simulink model "WindPrototipeN"  (R2019b)
settings: Solver=ode23s  StartTime=0.0  StopTime=Ts  FixedStep=2  RelTol=5
values from neighbouring files (symbols this model uses):
  c1 = 0.51763    [matlab.mat]
  c2 = 116    [matlab.mat]
  c3 = 0.4    [matlab.mat]
  c4 = 5    [matlab.mat]
  c5 = 21    [matlab.mat]
  c6 = 0.006795    [matlab.mat]
  Tp = 2e-05    [matlab.mat]
undefined symbols (not defined in the file or in its folder): Cogent, DiscIntNeverNeededParam, Ion, Kepware, Lithium, localhost, sigbuilder_block
libraries: powerlib x266, powerlib_extras x83, simulink x30, powerlib_meascontrol x13, opclib x11, sldrtlib x8, electricdrivelib x3
(part 4 of 9)

== system WindPrototipeN/Дом 2/ПОТРЕБИТЕЛЬ1 ==
  1000 Вт1 : powerlib/Elements/Three-Phase Parallel RLC Load  LConnTagsString=A|B|C  Configuration=Y (grounded)  NominalVoltage=385  Vabc=[1e3 1e3 1e3]  Vabcp=[1e3 1e3 1e3]  NominalFrequency=50  UnbalancedPower=off  ActivePower=1000  InductivePower=0  CapacitivePower=0  Pabc=[10e3 9e3 11e3]  QLabc=[100 90 110]  QCabc=[100 90 110]  Pabcp=[10e3 9e3 11e3]  QLabcp=[100 90 110]  QCabcp=[100 90 110]  Measurements=None  LoadType=constant Z
      settings: SourceProductName=Simscape Electrical
  1500 Вт1 : powerlib/Elements/Three-Phase Parallel RLC Load  LConnTagsString=A|B|C  Configuration=Y (grounded)  NominalVoltage=385  Vabc=[1e3 1e3 1e3]  Vabcp=[1e3 1e3 1e3]  NominalFrequency=50  UnbalancedPower=off  ActivePower=1000  InductivePower=0  CapacitivePower=0  Pabc=[10e3 9e3 11e3]  QLabc=[100 90 110]  QCabc=[100 90 110]  Pabcp=[10e3 9e3 11e3]  QLabcp=[100 90 110]  QCabcp=[100 90 110]  Measurements=None  LoadType=constant Z
      settings: SourceProductName=Simscape Electrical
  500 Вт (1)1 : powerlib/Elements/Three-Phase Parallel RLC Load  LConnTagsString=A|B|C  Configuration=Y (grounded)  NominalVoltage=385  Vabc=[1e3 1e3 1e3]  Vabcp=[1e3 1e3 1e3]  NominalFrequency=50  UnbalancedPower=off  ActivePower=500  InductivePower=0  CapacitivePower=0  Pabc=[10e3 9e3 11e3]  QLabc=[100 90 110]  QCabc=[100 90 110]  Pabcp=[10e3 9e3 11e3]  QLabcp=[100 90 110]  QCabcp=[100 90 110]  Measurements=None  LoadType=constant Z
      settings: SourceProductName=Simscape Electrical
  500 Вт (2)1 : powerlib/Elements/Three-Phase Parallel RLC Load  LConnTagsString=A|B|C  Configuration=Y (grounded)  NominalVoltage=385  Vabc=[1e3 1e3 1e3]  Vabcp=[1e3 1e3 1e3]  NominalFrequency=50  UnbalancedPower=off  ActivePower=500  InductivePower=0  CapacitivePower=0  Pabc=[10e3 9e3 11e3]  QLabc=[100 90 110]  QCabc=[100 90 110]  Pabcp=[10e3 9e3 11e3]  QLabcp=[100 90 110]  QCabcp=[100 90 110]  Measurements=None  LoadType=constant Z
      settings: SourceProductName=Simscape Electrical
  BL : powerlib/Measurements/Three-Phase V-I Measurement  VoltageMeasurement=phase-to-ground  SetLabelV=on  LabelV=Vabc_BL_ex  Vpu=off  VpuLL=off  CurrentMeasurement=yes  SetLabelI=on  LabelI=Iabc_BL_ex  Ipu=off  Pbase=100e6  Vbase=500e3  OutputType=Magnitude  PhasorSimulation=off  PSBequivalent=0
      settings: SourceProductName=Simscape Electrical
  Subsystem1 : Subsystem
  Three-Phase Breaker10 : powerlib/Elements/Three-Phase Breaker  InitialState=open  SwitchA=on  SwitchB=on  SwitchC=on  SwitchTimes=[6 7]  External=on  BreakerResistance=0.001  SnubberResistance=1e6  SnubberCapacitance=inf  Measurements=None
      settings: SourceProductName=Simscape Electrical
  Three-Phase Breaker11 : powerlib/Elements/Three-Phase Breaker  InitialState=open  SwitchA=on  SwitchB=on  SwitchC=on  SwitchTimes=[7 10]  External=on  BreakerResistance=0.001  SnubberResistance=1e6  SnubberCapacitance=inf  Measurements=None
      settings: SourceProductName=Simscape Electrical
  Three-Phase Breaker8 : powerlib/Elements/Three-Phase Breaker  InitialState=open  SwitchA=on  SwitchB=on  SwitchC=on  SwitchTimes=[0 5]  External=on  BreakerResistance=0.001  SnubberResistance=1e6  SnubberCapacitance=inf  Measurements=None
      settings: SourceProductName=Simscape Electrical
  Three-Phase Breaker9 : powerlib/Elements/Three-Phase Breaker  InitialState=open  SwitchA=on  SwitchB=on  SwitchC=on  SwitchTimes=[2 5]  External=on  BreakerResistance=0.001  SnubberResistance=1e6  SnubberCapacitance=inf  Measurements=None
      settings: SourceProductName=Simscape Electrical
  Блок измерений : powerlib/Measurements/Three-Phase V-I Measurement  VoltageMeasurement=phase-to-ground  SetLabelV=off  LabelV=V1  Vpu=off  VpuLL=off  CurrentMeasurement=yes  SetLabelI=off  LabelI=I1  Ipu=off  Pbase=5.5e3  Vbase=385  OutputType=Magnitude  PhasorSimulation=off  PSBequivalent=0
      settings: SourceProductName=Simscape Electrical
  Терминал нагрузки : Scope  NumInputPorts=2
  A : PMIOPort  Side=Left
  B : PMIOPort  Port=2  Side=Left
  C : PMIOPort  Port=3  Side=Left
  tag scope: Iload_ex=global, Load2Home1=global, Load2Home2=global, Load2Home3=global, Load2Home4=global, Vload_ex=global
  wires:
  Блок измерений/1 -> [Vload_ex], Терминал нагрузки/1  "Напряжение, В"
  Блок измерений/2 -> [Iload_ex], Терминал нагрузки/2  "Сила тока, А"
  Subsystem1/3(Out3) -> [Load2Home3], Three-Phase Breaker10/1
  Subsystem1/1(Out1) -> [Load2Home1], Three-Phase Breaker8/1
  Subsystem1/4(Out4) -> [Load2Home4], Three-Phase Breaker11/1
  Subsystem1/2(Out2) -> [Load2Home2], Three-Phase Breaker9/1
  connections:
  BL/RConn1 -- Блок измерений/LConn1
  BL/RConn2 -- Блок измерений/LConn2
  BL/RConn3 -- Блок измерений/LConn3
  BL/LConn1 -- A/RConn1
  BL/LConn2 -- B/RConn1
  C/RConn1 -- BL/LConn3
  Three-Phase Breaker10/RConn1 -- Three-Phase Breaker9/RConn1 -- Блок измерений/RConn1 -- Three-Phase Breaker8/RConn1 -- Three-Phase Breaker11/RConn1
  Three-Phase Breaker10/RConn2 -- Three-Phase Breaker9/RConn2 -- Three-Phase Breaker8/RConn2 -- Блок измерений/RConn2 -- Three-Phase Breaker11/RConn2
  Three-Phase Breaker10/RConn3 -- Three-Phase Breaker9/RConn3 -- Three-Phase Breaker8/RConn3 -- Блок измерений/RConn3 -- Three-Phase Breaker11/RConn3
  500 Вт (1)1/LConn3 -- Three-Phase Breaker8/LConn3
  500 Вт (2)1/LConn2 -- Three-Phase Breaker9/LConn2
  1000 Вт1/LConn2 -- Three-Phase Breaker10/LConn2
  1500 Вт1/LConn3 -- Three-Phase Breaker11/LConn3
  1500 Вт1/LConn2 -- Three-Phase Breaker11/LConn2
  500 Вт (2)1/LConn1 -- Three-Phase Breaker9/LConn1
  1000 Вт1/LConn3 -- Three-Phase Breaker10/LConn3
  500 Вт (1)1/LConn2 -- Three-Phase Breaker8/LConn2
  1000 Вт1/LConn1 -- Three-Phase Breaker10/LConn1
  500 Вт (2)1/LConn3 -- Three-Phase Breaker9/LConn3
  1500 Вт1/LConn1 -- Three-Phase Breaker11/LConn1
  500 Вт (1)1/LConn1 -- Three-Phase Breaker8/LConn1

== system WindPrototipeN/Дом 2/СОЛНЕЧНЫЕ ПАНЕЛИ1 ==
  note: boost
  Солнечная радиация : Inport
  11*2=666 V : Subsystem
  FW Diode1 : powerlib/Power Electronics/Diode  Ron=0.01  Lon=0  Vf=0.8  IC=0  UseSnubber=off  Rs=100  Cs=0.1e-6  Measurements=off
      settings: SourceProductName=Simscape Electrical
  Gain : Gain  Gain=4732*2/1000
  IL1 : powerlib/Measurements/Current Measurement  PhasorSimulation=off  OutputType=Complex  PSBequivalent=0
      settings: SourceProductName=Simscape Electrical
  Mean Value1 : powerlib_extras/Measurements/Mean Value  Period=0.0045
      settings: SourceProductName=Simscape Electrical  SourceProductBaseCode=PS
  Mux : Mux  Inputs=2
  Product6 : Product  RndMeth=Zero
  Vdc2 : powerlib/Measurements/Voltage Measurement  Tag=PoWeRsYsTeMmEaSuReMeNt  PhasorSimulation=off  OutputType=Magnitude  PSBequivalent=0
      settings: SourceProductName=Simscape Electrical
  Мощность СП1 : Scope
  Мощность СП2 : Scope
  Мощность СП3_2 : Scope
  Мощность СП_2 : Scope
  Терминал данных параметров солнечной панели2 : Scope  NumInputPorts=4
  + : PMIOPort  Side=Right
  - : PMIOPort  Port=2  Side=Right
  Sp : Outport  VectorParamsAs1DForOutWhenUnconnected=off
  tag scope: Scur_ex=global, Sp_ex=global, Svol_ex=global
  wires:
  Vdc2/1 -> [Svol_ex], Мощность СП2/1, Терминал данных параметров солнечной панели2/4, Product6/1  "Напряжение, В"
  Product6/1 -> Mux/2, Sp/1, Терминал данных параметров солнечной панели2/2, [Sp_ex]  "Выходная мощность СЭУ, Вт"
  Gain/1 -> Mux/1, Терминал данных параметров солнечной панели2/1  "Интенсивность солнечной радиации, Вт/м2"
  Mux/1 -> Мощность СП_2/1
  Mean Value1/1 -> Product6/2
  IL1/1 -> Терминал данных параметров солнечной панели2/3, Mean Value1/1, [Scur_ex], Мощность СП1/1  "Сила тока, А"
  Солнечная радиация/1 -> Gain/1, Мощность СП3_2/1, 11*2=666 V/1(In1)
  connections:
  11*2=666 V/RConn2 -- Vdc2/LConn2 -- -/RConn1
  +/RConn1 -- IL1/RConn1
  11*2=666 V/RConn1 -- FW Diode1/LConn1 -- Vdc2/LConn1
  IL1/LConn1 -- FW Diode1/RConn1

== system WindPrototipeN/Дом 3/DC//AC 220В1 ==
  LC Фильтр : Subsystem
  PWM IGBT Inverter1 : powerlib/Power Electronics/Universal Bridge  Arms=3  SnubberResistance=5000  SnubberCapacitance=inf  Device=IGBT / Diodes  Ron=1e-3  Lon=0  ForwardVoltages="[  0.0  0.0  ]"  ForwardVoltage=.8  GTOparameters=[ 1e-6 ,1e-6 ]  IGBTparameters=[ 1e-6 , 2e-6 ]  Measurements=Device currents  Measurements_2=None  converterType=Rectifier
      settings: SourceProductName=Simscape Electrical
  Инвертор DC/AC : Subsystem
  Терминал инвертора : Scope  NumInputPorts=2
  A : PMIOPort  Side=Right
  B : PMIOPort  Port=2  Side=Right
  C : PMIOPort  Port=3  Side=Right
  + IGBT1 : PMIOPort  Port=4  Side=Left
  - IGBT1 : PMIOPort  Port=5  Side=Left
  wires:
  Инвертор DC/AC/3(Pulses) -> PWM IGBT Inverter1/1
  Инвертор DC/AC/1(VL) -> Терминал инвертора/1  "Напряжение на входе, В"
  Инвертор DC/AC/2(Vp) -> Терминал инвертора/2  "Напряжение от преобразователя, В"
  connections:
  LC Фильтр/LConn1 -- PWM IGBT Inverter1/LConn1
  LC Фильтр/RConn3 -- C/RConn1 -- Инвертор DC/AC/LConn1
  Инвертор DC/AC/LConn2 -- B/RConn1 -- LC Фильтр/RConn2
  LC Фильтр/RConn1 -- A/RConn1 -- Инвертор DC/AC/LConn3
  LC Фильтр/LConn3 -- PWM IGBT Inverter1/LConn3
  LC Фильтр/LConn2 -- PWM IGBT Inverter1/LConn2
  + IGBT1/RConn1 -- PWM IGBT Inverter1/RConn1
  - IGBT1/RConn1 -- PWM IGBT Inverter1/RConn2

== system WindPrototipeN/Дом 3/DC//DC ПРЕОБРАЗОВАТЕЛЬ ВЭУ1 ==
  Add : Sum
  CBus : powerlib/Elements/Series RLC Branch  LConnTagsString=__new0  RConnTagsString=__new0  BranchType=RC  Resistance=0.2  Inductance=1e-3  SetiL0=off  InitialCurrent=0  Capacitance=7500e-6  Setx0=on  InitialVoltage=100  Measurements=None
      settings: SourceProductName=Simscape Electrical
  Chopper : Subsystem  mask(SPSdrives Converter){SnubberResistance=10e3, SnubberCapacitance=inf, Ron=1e-3, ForwardVoltages=[1.3,1.3], IGBTParameters=[0,0], converterType=Inverter}
      mask prompts: SnubberResistance "Snubber resistance Rs (Ohms):"; SnubberCapacitance "Snubber capacitance Cs (F):"; Ron "Ron (Ohms):"; ForwardVoltages "Forward voltages [Device Vf(V), Diode Vd (V)]"; IGBTParameters "[Tf(s), Tt(s)]:"; converterType "Converter type:"
      mask help: This model implements an average-value buck converter."Duty Cycle" contains the duty cycle of the internal IGBT device.
      mask TypeOptions converterType: Rectifier | Inverter
      mask Display: plot(0,0,100,100,[39 39 23.8],[71 28 28],[44 56 49.6 56 52.8 56 61 61],[39.2 33.6 32.8 33.6 40.8 33.6 30 12.4],[44 44 44 61 61],[28 71 60 66.4 90],[75 67 83 75 67 83 75 75],[54 42 42 54 54 54 54 66],[61 75 75],[24 24 42],[75 75 61],[66,76,76])
  Constant : Constant  Value=100
  Current controller DISCRETE1 : Subsystem  mask(PI controller){Kp=0.0005, Ki=0.15, Ts=20e-6}
      mask prompts: Kp "Proportional gain (Kp)"; Ki "Integral gain (Ki)"; Ts "Sample time (s) :"
      mask help: Proportional-Integral Speed Controller
      mask Display: plot(0,0,100,100,[35,35,65],[70,30,30],[35,65],[45,60])
  Current controller DISCRETE2 : Subsystem  mask(PI controller){Kp=0.0005, Ki=0.15, Ts=20e-6}
      mask prompts: Kp "Proportional gain (Kp)"; Ki "Integral gain (Ki)"; Ts "Sample time (s) :"
      mask help: Proportional-Integral Speed Controller
      mask Display: plot(0,0,100,100,[35,35,65],[70,30,30],[35,65],[45,60])
  Duty Cycles : Subsystem
  IL2 : powerlib/Measurements/Current Measurement  PhasorSimulation=off  OutputType=Complex  PSBequivalent=0
      settings: SourceProductName=Simscape Electrical
  IL4 : powerlib/Measurements/Current Measurement  PhasorSimulation=off  OutputType=Complex  PSBequivalent=0
      settings: SourceProductName=Simscape Electrical
  L : powerlib/Elements/Series RLC Branch  LConnTagsString=__new0  RConnTagsString=__new0  BranchType=L  Resistance=0.3  Inductance=500e-6  SetiL0=off  InitialCurrent=0  Capacitance=100e-6  Setx0=off  InitialVoltage=0  Measurements=None
      settings: SourceProductName=Simscape Electrical
  Timer : Subsystem  DialogController=POWERSYS.PowerSysDialog  mask(Timer){t=[ 0  1], e=[1 1 ]}
      mask prompts: t "Time (s):"; e "Amplitude:"
      mask help:
      | Generates a signal changing at specified times.
      |
      | If a signal value is not specified at time zero, the output is kept at 0 until the first specified transition time.
      mask init: same as WindPrototipeN/Дом 1/DC//DC ПРЕОБРАЗОВАТЕЛЬ ВЭУ/Timer
      mask Help: web(psbhelp)
      mask Display: plot( tv(2:end-1), opv(2:end-1) )
  Voltage Measurement : powerlib/Measurements/Voltage Measurement  PhasorSimulation=off  OutputType=Complex  PSBequivalent=0
      settings: SourceProductName=Simscape Electrical
  Voltage Measurement1 : powerlib/Measurements/Voltage Measurement  PhasorSimulation=off  OutputType=Complex  PSBequivalent=0
      settings: SourceProductName=Simscape Electrical
  Диод : powerlib/Power Electronics/Diode  Ron=0.01  Lon=0  Vf=0.8  IC=0  UseSnubber=off  Rs=100  Cs=0.1e-6  Measurements=off
      settings: SourceProductName=Simscape Electrical
  Терминал вход : Scope  NumInputPorts=2
  Терминал выход boost DC/DC : Scope  NumInputPorts=2
  Фильтр : TransferFcn  Denominator=[0.001 1]
  Выход + : PMIOPort  Side=Right
  Вход - : PMIOPort  Port=2  Side=Left
  Выход - : PMIOPort  Port=3  Side=Right
  Вход + : PMIOPort  Port=4  Side=Left
  tag scope: WindDCoutA_ex_2=global, WindDCoutV_ex_2=global
  wires:
  Duty Cycles/1(dc) -> Chopper/1(Duty Cycle)
  Current controller DISCRETE2/1(Delta Ec) -> Add/2
  Current controller DISCRETE1/1(Ec) -> Add/1
  Voltage Measurement1/1 -> Терминал вход/1
  [Wp_ex_2] -> Current controller DISCRETE2/2(Ppv)
  IL4/1 -> [WindDCoutA_ex_2], Терминал выход boost DC/DC/2  "Сила тока, А"
  IL2/1 -> Терминал вход/2  "Сила тока, А"
  Add/1 -> Duty Cycles/1(Ec)
  Timer/1(Out) -> Current controller DISCRETE2/1(Pref)
  Voltage Measurement/1 -> [WindDCoutV_ex_2], Терминал выход boost DC/DC/1, Фильтр/1
  Constant/1 -> Current controller DISCRETE1/2(Uref)
  Фильтр/1 -> Current controller DISCRETE1/1(UBus)
  connections:
  Voltage Measurement1/LConn1 -- L/RConn1 -- IL2/RConn1
  Chopper/LConn2 -- Вход -/RConn1 -- Voltage Measurement1/LConn2 -- Voltage Measurement/LConn2 -- Выход -/RConn1 -- CBus/RConn1
  IL4/RConn1 -- Выход +/RConn1
  CBus/LConn1 -- IL4/LConn1 -- Voltage Measurement/LConn1 -- Chopper/LConn1
  Вход +/RConn1 -- Диод/LConn1
  Chopper/RConn1 -- L/LConn1
  Диод/RConn1 -- IL2/LConn1

== system WindPrototipeN/Дом 3/DC//DC ПРЕОБРАЗОВАТЕЛЬ СП1 ==
  Add : Sum
  CBus : powerlib/Elements/Series RLC Branch  LConnTagsString=__new0  RConnTagsString=__new0  BranchType=RC  Resistance=0.2  Inductance=1e-3  SetiL0=off  InitialCurrent=0  Capacitance=7500e-6  Setx0=on  InitialVoltage=100  Measurements=None
      settings: SourceProductName=Simscape Electrical
  Chopper : Subsystem  mask(SPSdrives Converter){SnubberResistance=10e3, SnubberCapacitance=inf, Ron=1e-3, ForwardVoltages=[1.3,1.3], IGBTParameters=[0,0], converterType=Inverter}
      mask prompts: SnubberResistance "Snubber resistance Rs (Ohms):"; SnubberCapacitance "Snubber capacitance Cs (F):"; Ron "Ron (Ohms):"; ForwardVoltages "Forward voltages [Device Vf(V), Diode Vd (V)]"; IGBTParameters "[Tf(s), Tt(s)]:"; converterType "Converter type:"
      mask help: This model implements an average-value buck converter."Duty Cycle" contains the duty cycle of the internal IGBT device.
      mask TypeOptions converterType: Rectifier | Inverter
      mask Display: plot(0,0,100,100,[39 39 23.8],[71 28 28],[44 56 49.6 56 52.8 56 61 61],[39.2 33.6 32.8 33.6 40.8 33.6 30 12.4],[44 44 44 61 61],[28 71 60 66.4 90],[75 67 83 75 67 83 75 75],[54 42 42 54 54 54 54 66],[61 75 75],[24 24 42],[75 75 61],[66,76,76])
  Constant : Constant  Value=100
  Current controller DISCRETE1 : Subsystem  mask(PI controller){Kp=0.0005, Ki=0.15, Ts=20e-6}
      mask prompts: Kp "Proportional gain (Kp)"; Ki "Integral gain (Ki)"; Ts "Sample time (s) :"
      mask help: Proportional-Integral Speed Controller
      mask Display: plot(0,0,100,100,[35,35,65],[70,30,30],[35,65],[45,60])
  Current controller DISCRETE2 : Subsystem  mask(PI controller){Kp=0.0005, Ki=0.15, Ts=20e-6}
      mask prompts: Kp "Proportional gain (Kp)"; Ki "Integral gain (Ki)"; Ts "Sample time (s) :"
      mask help: Proportional-Integral Speed Controller
      mask Display: plot(0,0,100,100,[35,35,65],[70,30,30],[35,65],[45,60])
  Duty Cycles : Subsystem
  IL2 : powerlib/Measurements/Current Measurement  PhasorSimulation=off  OutputType=Complex  PSBequivalent=0
      settings: SourceProductName=Simscape Electrical
  IL4 : powerlib/Measurements/Current Measurement  PhasorSimulation=off  OutputType=Complex  PSBequivalent=0
      settings: SourceProductName=Simscape Electrical
  L : powerlib/Elements/Series RLC Branch  LConnTagsString=__new0  RConnTagsString=__new0  BranchType=L  Resistance=0.3  Inductance=500e-6  SetiL0=off  InitialCurrent=0  Capacitance=100e-6  Setx0=off  InitialVoltage=0  Measurements=None
      settings: SourceProductName=Simscape Electrical
  Timer : Subsystem  DialogController=POWERSYS.PowerSysDialog  mask(Timer){t=[ 0  1], e=[1 1 ]}
      mask prompts: t "Time (s):"; e "Amplitude:"
      mask help:
      | Generates a signal changing at specified times.
      |
      | If a signal value is not specified at time zero, the output is kept at 0 until the first specified transition time.
      mask init: same as WindPrototipeN/Дом 1/DC//DC ПРЕОБРАЗОВАТЕЛЬ ВЭУ/Timer
      mask Help: web(psbhelp)
      mask Display: plot( tv(2:end-1), opv(2:end-1) )
  Voltage Measurement : powerlib/Measurements/Voltage Measurement  PhasorSimulation=off  OutputType=Complex  PSBequivalent=0
      settings: SourceProductName=Simscape Electrical
  Voltage Measurement1 : powerlib/Measurements/Voltage Measurement  PhasorSimulation=off  OutputType=Complex  PSBequivalent=0
      settings: SourceProductName=Simscape Electrical
  Диод : powerlib/Power Electronics/Diode  Ron=0.01  Lon=0  Vf=0.8  IC=0  UseSnubber=off  Rs=100  Cs=0.1e-6  Measurements=off
      settings: SourceProductName=Simscape Electrical
  Терминал вход : Scope  NumInputPorts=2
  Терминал выход boost DC/DC : Scope  NumInputPorts=2
  Фильтр : TransferFcn  Denominator=[0.001 1]
  Выход + : PMIOPort  Side=Right
  Выход - : PMIOPort  Port=2  Side=Right
  Вход + : PMIOPort  Port=3  Side=Left
  Вход - : PMIOPort  Port=4  Side=Left
  tag scope: SolarDCoutA_ex_2=global, SolarDCoutV_ex_2=global
  wires:
  Current controller DISCRETE2/1(Delta Ec) -> Add/2
  IL2/1 -> Терминал вход/2  "Сила тока, А"
  [Sp_ex_2] -> Current controller DISCRETE2/2(Ppv)
  IL4/1 -> [SolarDCoutA_ex_2], Терминал выход boost DC/DC/2  "Сила тока, А"
  Add/1 -> Duty Cycles/1(Ec)
  Current controller DISCRETE1/1(Ec) -> Add/1
  Voltage Measurement1/1 -> Терминал вход/1
  Timer/1(Out) -> Current controller DISCRETE2/1(Pref)
  Constant/1 -> Current controller DISCRETE1/2(Uref)
  Duty Cycles/1(dc) -> Chopper/1(Duty Cycle)
  Фильтр/1 -> Current controller DISCRETE1/1(UBus)
  Voltage Measurement/1 -> [SolarDCoutV_ex_2], Терминал выход boost DC/DC/1, Фильтр/1
  connections:
  CBus/LConn1 -- Chopper/LConn1 -- IL4/LConn1 -- Voltage Measurement/LConn1
  Выход -/RConn1 -- Voltage Measurement/LConn2 -- Chopper/LConn2 -- Voltage Measurement1/LConn2 -- Вход -/RConn1 -- CBus/RConn1
  IL2/RConn1 -- Voltage Measurement1/LConn1 -- L/RConn1
  IL4/RConn1 -- Выход +/RConn1
  Chopper/RConn1 -- L/LConn1
  Диод/RConn1 -- IL2/LConn1
  Вход +/RConn1 -- Диод/LConn1

== system WindPrototipeN/Дом 3/MPPT КОНТРОЛЛЕР МОЩНОСТИ ВЭУ1 ==
  Wm : Inport
  Id : Inport  Port=2
  Vd : Inport  Port=3
  Unit Delay3 : UnitDelay  SampleTime=-1  HasFrameUpgradeWarning=on
  Биполярный транзистор (Chopper) : powerlib/Power Electronics/IGBT  Ron=0.001  Lon=0  Vf=1  Tf=1e-6  Tt=2e-6  IC=0  Rs=1e5  Cs=inf  Measurements=off
      settings: SourceProductName=Simscape Electrical
  Контроллер силы тока : Subsystem  mask{h=0.1}
      mask prompts: h "Hysteresis band (A)"
      mask help: Hysteresis Current Controller
      mask Display: plot(0,0,100,100,[45,45],[35,65],[55,55],[35,65],[45,65],[65,65],[35,55],[35,35])
  Расчет опорного момента : Subsystem
  Расчет опорной силы тока : Subsystem
  Терминал ошибки : Scope  NumInputPorts=2
  Фильтр : powerlib_extras/Discrete  Control Blocks/Discrete 1st-Order Filter  FilterType=Lowpass  Tc=100e-3  Ts=20e-6  Initialize=off  Vac_Init=[0.8 -25 60]  Vdc_Init=-0.4  PlotResponse=off  param1=[1 500 0.1]
      settings: SourceProductName=Simscape Electrical  SourceProductBaseCode=PS
  - : PMIOPort  Side=Right
  + : PMIOPort  Port=2  Side=Left
  wires:
  Id/1 -> Unit Delay3/1
  Расчет опорной силы тока/1(Id_ref) -> Фильтр/1
  Расчет опорного момента/1(Tref) -> Расчет опорной силы тока/1(Tref)
  Wm/1 -> Расчет опорного момента/1(wm), Расчет опорной силы тока/2(wm)
  Контроллер силы тока/1(g) -> Биполярный транзистор (Chopper)/1, Терминал ошибки/1
  Фильтр/1 -> Контроллер силы тока/1(Iref)
  Контроллер силы тока/2(error1) -> Терминал ошибки/2
  Vd/1 -> Расчет опорной силы тока/3(Vd)
  Unit Delay3/1 -> Контроллер силы тока/2(Ia)
  connections:
  Биполярный транзистор (Chopper)/LConn1 -- +/RConn1
  Биполярный транзистор (Chopper)/RConn1 -- -/RConn1

== system WindPrototipeN/Дом 3/PRE_Home1 ==
  Add : Sum
  Discrete Mean value1 : powerlib_extras/Discrete Measurements/Discrete  Mean value  Freq=50  Vinit=0  Ts=20e-6
      settings: SourceProductName=Simscape Electrical  SourceProductBaseCode=PS
  tag scope: PRE_ex_3=global
  wires:
  Discrete Mean value1/1 -> [PRE_ex_3]
  Add/1 -> Discrete Mean value1/1
  [Sp_ex_2] -> Add/1
  [Wp_ex_2] -> Add/2

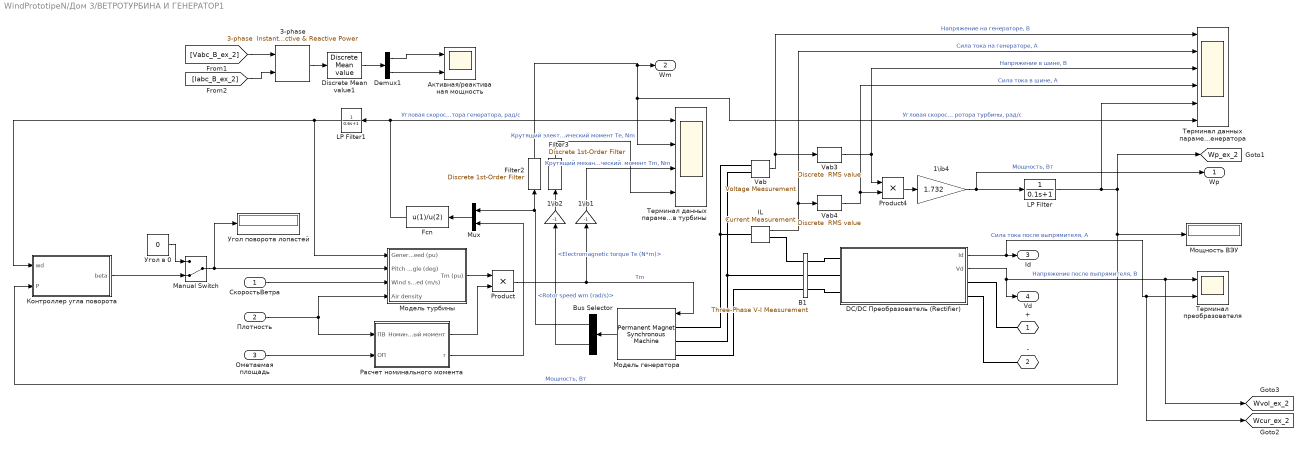
== system WindPrototipeN/Дом 3/ВЕТРОТУРБИНА И ГЕНЕРАТОР1 ==
  СкоростьВетра : Inport
  Плотность : Inport  Port=2
  Ометаемая площадь : Inport  Port=3
  1\ib1 : Gain  Gain=-1  SaturateOnIntegerOverflow=on  OutDataTypeStr=Inherit: Same as input  ParamDataTypeStr=Inherit: Same as input
  1\ib2 : Gain  Gain=-1  SaturateOnIntegerOverflow=on  OutDataTypeStr=Inherit: Same as input  ParamDataTypeStr=Inherit: Same as input
  1\ib4 : Gain  Gain=1.732  SaturateOnIntegerOverflow=on  OutDataTypeStr=Inherit: Same as input  ParamDataTypeStr=Inherit: Same as input
  "3-phase " : powerlib_extras/Measurements/3-phase  Instantaneous  Active & Reactive Power
      settings: SourceProductName=Simscape Electrical  SourceProductBaseCode=PS
  B1 : powerlib/Measurements/Three-Phase V-I Measurement  VoltageMeasurement=phase-to-ground  SetLabelV=on  LabelV=Vabc_B_ex_2  Vpu=off  VpuLL=off  CurrentMeasurement=yes  SetLabelI=on  LabelI=Iabc_B_ex_2  Ipu=off  Pbase=100e6  Vbase=500e3  OutputType=Magnitude  PhasorSimulation=off  PSBequivalent=0
      settings: SourceProductName=Simscape Electrical
  Bus Selector : BusSelector  OutputSignals=Rotor speed wm (rad/s),Electromagnetic torque Te (N*m)
  DC/DC Преобразователь (Rectifier) : Subsystem
  Demux1 : Demux  Outputs=2
  Discrete Mean value1 : powerlib_extras/Discrete Measurements/Discrete  Mean value  Freq=50  Vinit=0  Ts=20e-6
      settings: SourceProductName=Simscape Electrical  SourceProductBaseCode=PS
  Fcn : Fcn  Expr=u(1)/u(2)
  Filter2 : powerlib_extras/Discrete  Control Blocks/Discrete 1st-Order Filter  FilterType=Lowpass  Tc=1e-3  Ts=20e-6  Initialize=off  Vac_Init=[0.8 -25 60]  Vdc_Init=-0.4  PlotResponse=off  param1=[1 500 0.1]
      settings: SourceProductName=Simscape Electrical  SourceProductBaseCode=PS
  Filter3 : powerlib_extras/Discrete  Control Blocks/Discrete 1st-Order Filter  FilterType=Lowpass  Tc=1e-3  Ts=20e-6  Initialize=off  Vac_Init=[0.8 -25 60]  Vdc_Init=-0.4  PlotResponse=off  param1=[1 500 0.1]
      settings: SourceProductName=Simscape Electrical  SourceProductBaseCode=PS
  IL : powerlib/Measurements/Current Measurement  PhasorSimulation=off  OutputType=Complex  PSBequivalent=0
      settings: SourceProductName=Simscape Electrical
  LP Filter : TransferFcn  Denominator=[0.1 1]
  LP Filter1 : TransferFcn  Denominator=[0.6 1]
  Manual Switch : ManualSwitch  CurrentSetting=0
  Mux : Mux  Inputs=2
  Product : Product  RndMeth=Zero
  Product4 : Product  RndMeth=Zero
  Vab : powerlib/Measurements/Voltage Measurement  PhasorSimulation=off  OutputType=Complex  PSBequivalent=0
      settings: SourceProductName=Simscape Electrical
  Vab3 : powerlib_extras/Discrete Measurements/Discrete  RMS value  Freq=50  Mag_Init=0  Ts=Tp
      settings: SourceProductName=Simscape Electrical  SourceProductBaseCode=PS
  Vab4 : powerlib_extras/Discrete Measurements/Discrete  RMS value  Freq=50  Mag_Init=0  Ts=Tp
      settings: SourceProductName=Simscape Electrical  SourceProductBaseCode=PS
  Активная/реактиваная мощность : Scope  NumInputPorts=2
  Контроллер угла поворота : Subsystem
  Модель генератора : powerlib/Machines/Permanent Magnet Synchronous Machine  NbPhases=3  FluxDistribution=Sinusoidal  RotorType=Salient-pole  MechanicalLoad=Torque Tm  PresetModel=No  ShowDetailedParameters=on  MeasurementBus=off  Resistance=0.425  Inductance=8.5e-3  dqInductances=[0.000835 0.000835]  La=0.000395  MachineConstant=Flux linkage established by magnets (V.s)  Flux=0.433  VoltageCst=471.2251  TorqueCst=3.897  Flat=120  Mechanical=[0.0119 0.0011 6]  PolePairs=5  InitialConditions=[0,0, 0,0]  InitialConditions5ph=[0 0 0 0 0 0]  RefAngle=90 degrees behind phase A axis (modified Park)  IterativeDiscreteModel=Trapezoidal non iterative  TsBlock=-1  TsPowergui=0
  Модель турбины : Subsystem  AncestorBlock=DRlib/Wind Generation/Wind Turbine  DialogController=POWERSYS.PowerSysDialog  mask(Wind Turbine){Pnom=8.5e3, Pelec_base=8.5e3/0.9, wind_base=10, P_wind_base=0.8, speed_nom=1, pitch_angle=0, DisplayTurbChar=off, c1_c6=[0.51763          116          0.4            5           21     0.006795], cp_nom=0.48, lambda_nom=8.1}
      mask prompts: Pnom "Nominal mechanical output power (W):"; Pelec_base "Base power of the electrical generator (VA):"; wind_base "Base wind speed (m/s):"; P_wind_base "Maximum power at base wind speed (pu of nominal mechanical power):"; speed_nom "Base rotational speed (p.u. of base generator speed):"; pitch_angle "Pitch angle beta to display wind-turbine power characteristics (beta >=0)  (deg):"; DisplayTurbChar "Display wind turbine power characteristics"
      mask help:
      | This block implements a variable pitch wind turbine model. The performance coefficient Cp of the turbine is the mechanical output power of the turbine divided by wind power and a function of wind speed, rotational speed, and pitch angle (beta). Cp reaches its maximum value at zero beta. Select the wind-turbine power characteristics display to plot the turbine characteristics at the specified pitch angle.
      |
      | The first input is the generator speed in per unit of the generator base speed. For a synchronous or asynchronous generator, the base speed is the synchronous speed. For a permanent-magnet generator, the base speed is defined as the speed producing nominal voltage at  no load. The second input is the blade pitch angle (beta) in degrees. The third input is the wind speed in m/s.
      |
      | The output is the torque applied to the generator shaft in per unit of the generator ratings.
      |
      | The turbine inertia must be added to the generator inertia.
      mask init: same as WindPrototipeN/Дом 1/ВЕТРОТУРБИНА И ГЕНЕРАТОР/Модель турбины
      mask Help: web(psbhelp);
      mask Callback Pnom:
      | ParVisible={'on','on','on','on','on','on','on','off','off','off',};
      | set_param(gcb,'MaskVisibilities',ParVisible);
      | c1_c6=str2num(get_param(gcb,'c1_c6'));
      | c1=c1_c6(1);c2=c1_c6(2);c3=c1_c6(3);c4=c1_c6(4);c5=c1_c6(5);c6=c1_c6(6);
      mask Callback DisplayTurbChar:
      | DisplayTurbChar=get_param(gcb,'DisplayTurbChar');
      | 
      | if strcmp(DisplayTurbChar,'on')
      |     fig_num=figure;
      | 	clf(fig_num);
      | 	[speed_nom,wind_base,P_wind_base,pitch_angle]=getSPSmaskvalues(gcb,{'speed_nom','wind_base','P_wind_base','pitch_angle'});
      | 	[c1_c6,lambda_nom,cp_nom]=getSPSmaskvalues(gcb,{'c1_c6','lambda_nom','cp_nom'});
      | 	c1=c1_c6(1);c2=c1_c6(2);c3=c1_c6(3);c4=c1_c6(4);c5=c1_c6(5);c6=c1_c6(6);
      | 
      | 	%Wind turbine typical characteristic data
      |     %c2=116;c3=0.4;c4=5;c5=21;
      |     %Computation of c1 and c6 for lambda_nom et cpmax
      |     %lambda_nom=8.1;
      |     %cp_max=0.48;
      |     %cp_nom=cp_max;
      | 
      |     %lambda_i_nom=1/(1/lambda_nom-0.035);
      |     %k_nom=-(c2*c5/lambda_i_nom-c4*c5-c2)*exp(-c5/lambda_i_nom)/lambda_nom^2;
      |     %c1=cp_max/((c2/lambda_i_nom-c4)*exp(-c5/lambda_i_nom)+k_nom*lambda_nom);
      |     %c6=k_nom*c1;
      | 
      | 	wr_elec_pu=1e-3:0.01:1.5;;
      |     wr_mec_pu=wr_elec_pu/speed_nom;
      |     wind_max=ceil((1.2/P_wind_base)^(1/3)*wind_base);
      |     wind_min=round(((0.1)/P_wind_base)^(1/3)*wind_base);
      |     wind1=wind_min:(wind_base-wind_min)/5:wind_base;
      |     wind2=wind_base+(wind_base-wind_min)/5:(wind_base-wind_min)/5:wind_max;
      |     wind_pu=[wind1 wind2]/wind_base;
      | 
      |     for k=1:length(wind_pu)
      |         for i=1:length(wr_mec_pu);
      |             lambda_pu=wr_mec_pu(i)/wind_pu(k);
      |             lambda=lambda_pu*lambda_nom;
      |             lambda_i=1/(1/(lambda+0.08*pitch_angle)-0.035/(pitch_angle^3+1));
      |             cp=c1*(c2/lambda_i-c3*pitch_angle-c4)*exp(-c5/lambda_i)+c6*lambda;
      |             cp_pu=cp/cp_nom;
      |             Pwind_pu(k,i)=wind_pu(k)^3*cp_pu*P_wind_base;
      |         end
      |     end
      |     for k=1:length(wind_pu)
      |         plot(wr_elec_pu,Pwind_pu(k,:))
      |         hold on
      |     end
      | 
      |     plot([speed_nom,speed_nom,0],[0,P_wind_base,P_wind_base],'r--')
      |     text(speed_nom+0.01,0+0.05,sprintf('%0.4g pu',speed_nom))
      |     text(0.01,P_wind_base+0.05,sprintf('Max. power at base wind speed (%0.4g m/s) and beta = 0 deg',wind_base))
      |     for i=1:length(wind_pu),
      |         p_max(i)=max(Pwind_pu(i,:));
      |         speed(i)=wr_elec_pu(find(Pwind_pu(i,:)==p_max(i)));
      |         text(speed(i),p_max(i),sprintf('%0.4g m/s',wind_pu(i)*wind_base))
      |     end
      |     plot([0 max(wr_elec_pu)],[0 0],'--')
      | 
      |     xlabel('Turbine speed (pu of nominal generator speed)')
      |     ylabel('Turbine output power (pu of nominal mechanical power)')
      |     title(sprintf('Turbine Power Characteristics (Pitch angle beta = %0.4g deg)',pitch_angle))
      |     axis([0 max(wr_elec_pu) min(Pwind_pu(1,:)) max(P_wind_base+0.1,max(wind_pu)^3*P_wind_base+0.1)])
      |     set_param(gcb,'DisplayTurbChar','off')
      | end
      mask Display: disp('');
  Мощность ВЭУ : Display
      settings: SampleTime=1e-3
  Расчет номинального момента : Subsystem
  Терминал данных параметров генератора : Scope  NumInputPorts=6
  Терминал данных параметров турбины : Scope  NumInputPorts=4
  Терминал преобразователя : Scope  NumInputPorts=2
  "Угол в 0 " : Constant  Value=0
  Угол поворота лопастей : Display
  + : PMIOPort  Tag=PMCPort  Side=Right
  - : PMIOPort  Tag=PMCPort  Port=2  Side=Right
  Wp : Outport  VectorParamsAs1DForOutWhenUnconnected=off
  Wm : Outport  Port=2  VectorParamsAs1DForOutWhenUnconnected=off
  Id : Outport  Port=3  VectorParamsAs1DForOutWhenUnconnected=off
  Vd : Outport  Port=4  VectorParamsAs1DForOutWhenUnconnected=off
  tag scope: Wcur_ex_2=global, Wp_ex_2=global, Wvol_ex_2=global
  wires:
  Модель турбины/1(Tm (pu)) -> Product/1
  Vab/1 -> Терминал данных параметров генератора/1, Vab3/1  "Напряжение на генераторе, В"
  IL/1 -> Терминал данных параметров генератора/2, Vab4/1  "Сила тока на генераторе, А"
  Product4/1 -> 1\ib4/1
  Product/1 -> Модель генератора/1, 1\ib1/1  "Tm"
  Vab3/1 -> Терминал данных параметров генератора/3, Product4/1  "Напряжение в шине, В"
  Vab4/1 -> Терминал данных параметров генератора/4, Product4/2  "Сила тока в шине, А"
  1\ib4/1 -> LP Filter/1, Wp/1  "Мощность, Вт"
  Модель генератора/1 -> Bus Selector/1
  Bus Selector/2 -> 1\ib2/1  "<Electromagnetic torque Te (N*m)>"
  1\ib2/1 -> Filter3/1
  Filter3/1 -> Терминал данных параметров турбины/4  "Крутящий электрический момент Te, Nm"
  1\ib1/1 -> Терминал данных параметров турбины/3  "Крутящий механический  момент Tm, Nm"
  СкоростьВетра/1 -> Модель турбины/3(Wind speed (m/s))
  Плотность/1 -> Модель турбины/4(Air density), Расчет номинального момента/1(ПВ)
  Ометаемая площадь/1 -> Расчет номинального момента/2(ОП)
  Расчет номинального момента/1(Номинальный момент) -> Product/2
  Mux/1 -> Fcn/1
  Расчет номинального момента/2(r) -> Mux/2
  Bus Selector/1 -> Filter2/1, Mux/1  "<Rotor speed wm (rad/s)>"
  Filter2/1 -> Терминал данных параметров генератора/6, Терминал данных параметров турбины/2, Wm/1  "Угловая скорость ротора турбины, рад/с"
  Manual Switch/1 -> Угол поворота лопастей/1, Модель турбины/2(Pitch angle (deg))
  [Iabc_B_ex_2] -> "3-phase "/2
  Demux1/1 -> Активная/реактиваная мощность/1
  [Vabc_B_ex_2] -> "3-phase "/1
  Discrete Mean value1/1 -> Demux1/1
  Demux1/2 -> Активная/реактиваная мощность/2
  "3-phase "/1 -> Discrete Mean value1/1
  LP Filter/1 -> Контроллер угла поворота/2(P), Мощность ВЭУ/1, [Wp_ex_2], Терминал данных параметров генератора/5  "Мощность, Вт"
  Fcn/1 -> LP Filter1/1, Терминал данных параметров турбины/1  "Угловая скорость ротора генератора, рад/с"
  Контроллер угла поворота/1(beta) -> Manual Switch/2
  "Угол в 0 "/1 -> Manual Switch/1
  LP Filter1/1 -> Контроллер угла поворота/1(wd), Модель турбины/1(Generator speed (pu))
  DC/DC Преобразователь (Rectifier)/2(Vd) -> [Wvol_ex_2], Терминал преобразователя/1, Vd/1  "Напряжение после выпрямителя, В"
  DC/DC Преобразователь (Rectifier)/1(Id) -> [Wcur_ex_2], Терминал преобразователя/2, Id/1  "Сила тока после выпрямителя, А"
  connections:
  Vab/LConn2 -- B1/LConn2 -- Модель генератора/LConn2
  Модель генератора/LConn3 -- B1/LConn3
  Vab/LConn1 -- Модель генератора/LConn1 -- IL/LConn1
  IL/RConn1 -- B1/LConn1
  DC/DC Преобразователь (Rectifier)/RConn1 -- +/RConn1
  B1/RConn1 -- DC/DC Преобразователь (Rectifier)/LConn1
  B1/RConn2 -- DC/DC Преобразователь (Rectifier)/LConn2
  DC/DC Преобразователь (Rectifier)/RConn2 -- -/RConn1
  DC/DC Преобразователь (Rectifier)/LConn3 -- B1/RConn3

== system WindPrototipeN/Дом 3/ВХОДНЫЕ ЗНАЧЕНИЯ ДЛЯ ВЭУ1 ==
  Скорость ветра (1-4) : Inport
  Плостность воздуха и температура (1-4) : Inport  Port=2
  Math Function3 : Math  Operator=square  SaturateOnIntegerOverflow=on
  Ramp : simulink/Sources/Ramp  slope=20  start=0  InitialOutput=0
  Saturation : Saturate  UpperLimit=12  LowerLimit=0
  Speed2 : powerlib_extras/Control  Blocks/Timer  t=[0 2 3.5]  e=[8 15 15]
      settings: SourceProductName=Simscape Electrical  SourceProductBaseCode=PS
  Задание кривой скорости : Subsystem  Tag=STV Subsys  LoadFcn=sigbuilder_block('load');  StartFcn=sigbuilder_block('start');  StopFcn=sigbuilder_block('stop');  ClipboardFcn=sigbuilder_block('clipboard');  mask(Sigbuilder block){tuvar=[0:10]}
      mask help: Simulink:masks:SigbuilderBlock_MD
      mask init:
      | if ~strcmp(get_param(bdroot(gcbh),'SimulationStatus'),'stopped') tuvar = sigbuilder_block('maskInit'); end
      settings: CopyFcn=sigbuilder_block('copy');  DeleteFcn=sigbuilder_block('delete');  ModelCloseFcn=sigbuilder_block('modelClose');  PreSaveFcn=sigbuilder_block('preSave');  PauseFcn=sigbuilder_block('pause');  ContinueFcn=sigbuilder_block('continue');  NameChangeFcn=sigbuilder_block('namechange');  OpenFcn=sigbuilder_block('open',[142.5 191.25 550.5 399.75 ]);  CloseFcn=sigbuilder_block('close');
      mask Display: plot(0, 0, 100, 100,[2, 2, 32, 32, 2], [68, 8, 8, 68, 68],[32, 2], [38, 38], [32, 19, 2],[53, 60, 44], [32, 17, 17, 2],[16, 16, 31, 31]);txt = getActiveGroup(gcbh);text(2, 100, txt,'verticalAlignment', 'top');
  Задание кривой скорости1 : Subsystem  Tag=STV Subsys  LoadFcn=sigbuilder_block('load');  StartFcn=sigbuilder_block('start');  StopFcn=sigbuilder_block('stop');  ClipboardFcn=sigbuilder_block('clipboard');  mask(Sigbuilder block){tuvar=[0:10]}
      mask help: Simulink:masks:SigbuilderBlock_MD
      mask init:
      | if ~strcmp(get_param(bdroot(gcbh),'SimulationStatus'),'stopped') tuvar = sigbuilder_block('maskInit'); end
      settings: CopyFcn=sigbuilder_block('copy');  DeleteFcn=sigbuilder_block('delete');  ModelCloseFcn=sigbuilder_block('modelClose');  PreSaveFcn=sigbuilder_block('preSave');  PauseFcn=sigbuilder_block('pause');  ContinueFcn=sigbuilder_block('continue');  NameChangeFcn=sigbuilder_block('namechange');  OpenFcn=sigbuilder_block('open',[142.5 191.25 550.5 399.75 ]);  CloseFcn=sigbuilder_block('close');
      mask Display: plot(0, 0, 100, 100,[2, 2, 32, 32, 2], [68, 8, 8, 68, 68],[32, 2], [38, 38], [32, 19, 2],[53, 60, 44], [32, 17, 17, 2],[16, 16, 31, 31]);txt = getActiveGroup(gcbh);text(2, 100, txt,'verticalAlignment', 'top');
  Пи : Gain  Gain=pi
  Плотность воздуха : MultiPortSwitch  Inputs=4
  "Плотность воздуха, +35С" : Constant  Value=1.1308
  "Плотность воздуха, -10C" : Constant  Value=1.3413
  "Плотность воздуха, 0C" : Constant  Value=1.2920
  "Плотность воздуха, 15C" : Constant  Value=1.2250
  Плотность воздуха1 : MultiPortSwitch  Inputs=4
  Радуис : Constant  Value=2.5
  Выход скорость ветра : Outport  OutDataTypeStr=double  VectorParamsAs1DForOutWhenUnconnected=off
  Выход плотность и температура воздуха : Outport  Port=2  VectorParamsAs1DForOutWhenUnconnected=off
  Ометаемая площадь : Outport  Port=3  VectorParamsAs1DForOutWhenUnconnected=off
  tag scope: WindSpeed_ex_2=global
  wires:
  Скорость ветра (1-4)/1 -> Плотность воздуха1/1
  "Плотность воздуха, 0C"/1 -> Плотность воздуха/3
  "Плотность воздуха, +35С"/1 -> Плотность воздуха/5
  "Плотность воздуха, 15C"/1 -> Плотность воздуха/2
  Радуис/1 -> Math Function3/1
  "Плотность воздуха, -10C"/1 -> Плотность воздуха/4
  Math Function3/1 -> Пи/1
  Задание кривой скорости/1(Signal 1) -> Плотность воздуха1/2
  Плостность воздуха и температура (1-4)/1 -> Плотность воздуха/1
  Плотность воздуха/1 -> Выход плотность и температура воздуха/1
  Пи/1 -> Ометаемая площадь/1
  Saturation/1 -> Плотность воздуха1/4  "Скорость ветра"
  Speed2/1 -> Плотность воздуха1/5  "Скорость ветра"
  Ramp/1 -> Saturation/1
  Плотность воздуха1/1 -> [WindSpeed_ex_2], Выход скорость ветра/1
  Задание кривой скорости1/1(Signal 1) -> Плотность воздуха1/3

== system WindPrototipeN/Дом 3/ВХОДНЫЕ ЗНАЧЕНИЯ ДЛЯ СЭС1 ==
  Номер (1,2) : Inport
  Задание кривой солнечной радиации : Subsystem  Tag=STV Subsys  LoadFcn=sigbuilder_block('load');  StartFcn=sigbuilder_block('start');  StopFcn=sigbuilder_block('stop');  ClipboardFcn=sigbuilder_block('clipboard');  mask(Sigbuilder block){tuvar=[0:10]}
      mask help: Simulink:masks:SigbuilderBlock_MD
      mask init:
      | if ~strcmp(get_param(bdroot(gcbh),'SimulationStatus'),'stopped') tuvar = sigbuilder_block('maskInit'); end
      settings: CopyFcn=sigbuilder_block('copy');  DeleteFcn=sigbuilder_block('delete');  ModelCloseFcn=sigbuilder_block('modelClose');  PreSaveFcn=sigbuilder_block('preSave');  PauseFcn=sigbuilder_block('pause');  ContinueFcn=sigbuilder_block('continue');  NameChangeFcn=sigbuilder_block('namechange');  OpenFcn=sigbuilder_block('open',[274.5 202.5 550.5 399.75 ]);  CloseFcn=sigbuilder_block('close');
      mask Display: plot(0, 0, 100, 100,[2, 2, 32, 32, 2], [68, 8, 8, 68, 68],[32, 2], [38, 38], [32, 19, 2],[53, 60, 44], [32, 17, 17, 2],[16, 16, 31, 31]);txt = getActiveGroup(gcbh);text(2, 100, txt,'verticalAlignment', 'top');
  Интенсивность солнечной радиации : Constant  Value=1000  SampleTime=20e-6
  Солнечная радиация : MultiPortSwitch  Inputs=2
  Интенсивность солнечной радиации : Outport  VectorParamsAs1DForOutWhenUnconnected=off
  tag scope: SolarRad_ex_2=global
  wires:
  Солнечная радиация/1 -> [SolarRad_ex_2], Интенсивность солнечной радиации/1
  Номер (1,2)/1 -> Солнечная радиация/1
  Задание кривой солнечной радиации/1(Signal 1) -> Солнечная радиация/2
  Интенсивность солнечной радиации/1 -> Солнечная радиация/3

== system WindPrototipeN/Дом 3/КОНТРОЛЛЕР БАТАРЕИ ==
  Vdc : Inport
  SOC. % : Inport  Port=2
  Ibat : Inport  Port=3
  Constant : Constant  Value=640
  Constant1 : Constant  Value=.8
  Constant3 : Constant
  Constant4 : Constant  Value=.8
  Data Type Conversion : DataTypeConversion  OutDataTypeStr=boolean  RndMeth=Simplest  SaturateOnIntegerOverflow=on
  Discrete PI Controller : Subsystem  AncestorBlock=|  DialogController=POWERSYS.PowerSysDialog  mask(Discrete PI Controller){Kp=2, Ki=120, Par_Limits=[100  -100], Init=0, Ts=2e-5}
      | powerlib_extras/Discrete 
      | Control Blocks/Discrete
      | PI Controller
      mask prompts: Kp "Proportional gain (Kp):"; Ki "Integral gain (Ki):"; Par_Limits "Output limits: [ Upper   Lower ]"; Init "Output initial value:"; Ts "Sample time:"
      mask help: This block implements a discrete PI controller.
      mask init:
      | UpperLimit=Par_Limits(1);
      | LowerLimit=Par_Limits(2);
      | power_initmask();
      mask Help: This block is part of a subset of blocks in the Extras library that does not have documentation associated with it, other than the block mask description.
      mask Display: disp('PI');
  Discrete PI Controller1 : Subsystem  AncestorBlock=|  DialogController=POWERSYS.PowerSysDialog  mask(Discrete PI Controller){Kp=60, Ki=550, Par_Limits=[1  -1], Init=0, Ts=2e-5}
      | powerlib_extras/Discrete 
      | Control Blocks/Discrete
      | PI Controller
      mask prompts: Kp "Proportional gain (Kp):"; Ki "Integral gain (Ki):"; Par_Limits "Output limits: [ Upper   Lower ]"; Init "Output initial value:"; Ts "Sample time:"
      mask help: This block implements a discrete PI controller.
      mask init:
      | UpperLimit=Par_Limits(1);
      | LowerLimit=Par_Limits(2);
      | power_initmask();
      mask Help: This block is part of a subset of blocks in the Extras library that does not have documentation associated with it, other than the block mask description.
      mask Display: disp('PI');
  Gain : Gain  Gain=1/640  SaturateOnIntegerOverflow=on  OutDataTypeStr=Inherit: Same as input  ParamDataTypeStr=Inherit: Same as input
  Gain1 : Gain  Gain=1/100  SaturateOnIntegerOverflow=on  OutDataTypeStr=Inherit: Same as input  ParamDataTypeStr=Inherit: Same as input
  Gain2 : Gain  Gain=1/100  SaturateOnIntegerOverflow=on  OutDataTypeStr=Inherit: Same as input  ParamDataTypeStr=Inherit: Same as input
  Logical Operator2 : Logic
  Logical Operator3 : Logic  Operator=NOT
  Math Function : Math  Operator=reciprocal  SignedPower=off  SaturateOnIntegerOverflow=on
  Mux : Mux  Inputs=2
  Mux1 : Mux  Inputs=2
  Product : Product
  Product2 : Product  RndMeth=Zero
  Ramp_generator : Subsystem
  Relational Operator : RelationalOperator  RndMeth=Nearest  InputSameDT=on
  Relational Operator1 : RelationalOperator  Operator=<=  RndMeth=Nearest  InputSameDT=on
  Relational Operator3 : RelationalOperator  Operator=>  RndMeth=Nearest  InputSameDT=on
  Relay : Relay  OnSwitchValue=2  OffSwitchValue=-2  OutDataTypeStr=Inherit: Inherit via back propagation
  Scope1 : Scope  NumInputPorts=2
  Scope2 : Scope  NumInputPorts=3
  Scope3 : Scope  NumInputPorts=4
  Scope4 : Scope  NumInputPorts=3
  Scope5 : Scope  NumInputPorts=2
  Sum : Sum  Inputs=+-  SaturateOnIntegerOverflow=on  InputSameDT=on  OutDataTypeStr=Inherit: Same as first input
  Sum1 : Sum  Inputs=|+-  InputSameDT=on
  Sum2 : Sum  Inputs=|+-  SaturateOnIntegerOverflow=on  InputSameDT=on  OutDataTypeStr=Inherit: Same as first input
  Переключатель S1 : Outport  VectorParamsAs1DForOutWhenUnconnected=off
  Переключатель S2 : Outport  Port=2  VectorParamsAs1DForOutWhenUnconnected=off
  Затвор : Outport  Port=3  VectorParamsAs1DForOutWhenUnconnected=off
  wires:
  Discrete PI Controller/1(Out) -> Sum1/1  "Выход ПИ-регулятора"
  Sum/1 -> Discrete PI Controller/1(Error)
  Vdc/1 -> Sum/2, Mux/2, Product/1  "Измеренное напряжение"
  Relay/1 -> Data Type Conversion/1
  Ibat/1 -> Sum1/2
  Sum1/1 -> Scope1/2, Relay/1  "Выход ПИ-регулятора"
  Gain1/1 -> Relational Operator1/1
  SOC. %/1 -> Gain1/1, Gain2/1  "Уровень заряда"
  Relational Operator1/1 -> Product2/2  "Если SOC <= 80%"
  Constant1/1 -> Relational Operator1/2
  Logical Operator3/1 -> Product2/1
  Product2/1 -> Переключатель S2/1, Scope5/1, Scope4/2, Scope3/1  "Логический выход S2"
  Relational Operator/1 -> Logical Operator2/1  "Условие"
  Constant3/1 -> Mux1/1, Sum2/2
  Sum2/1 -> Discrete PI Controller1/1(Error)  "Ошибка напряжение"
  Ramp_generator/1(ramp_out) -> Relational Operator/2  "Генератор"
  Discrete PI Controller1/1(Out) -> Scope2/2, Relational Operator/1  "Выход ПИ-регулятора напряжения"
  Relational Operator3/1 -> Logical Operator2/2, Scope3/3  "SOC > 80%"
  Gain2/1 -> Scope3/4, Relational Operator3/1  "SOC 100% -> 1"
  Constant4/1 -> Relational Operator3/2
  Logical Operator2/1 -> Scope2/3, Затвор/1  "Выход Gate"
  Mux/1 -> Scope1/1  "Напряжение на батареи, В (Uбат.уст = 640 В)"
  Mux1/1 -> Scope2/1  "Масштабированное напряжение, В (640 -> 1)"
  Data Type Conversion/1 -> Переключатель S1/1, Scope4/3, Scope5/2, Scope3/2, Logical Operator3/1  "Выход Gate"
  [BatCon_ex_3] -> Math Function/1, Sum/1, Mux/1
  Math Function/1 -> Product/2
  Product/1 -> Mux1/2, Sum2/1
